simulink model "config5sim_KinematicController_PosCon_H1N4_H2N3"  (R2019b)
settings: Solver=ode4  StartTime=0.0  StopTime=60  FixedStep=0.01  RelTol=1e-3  EnableMultiTasking=on
InitFcn:
  | U_Path
  | roboparam
  | W_init = W_i;
  | 
  | xref_min = min(x_ref);
  | xref_max = max(x_ref);
  | yref_min = min(y_ref);
  | yref_max = max(y_ref);
  | 
  | xQ_min = min(xQ);
  | xQ_max = max(xQ);
  | yQ_min = min(yQ);
  | yQ_max = max(yQ);
  | 
  | xref_rng = xref_max - xref_min;
  | yref_rng = yref_max - yref_min;
  | xQ_rng = (xQ_max - yQ_min);
  | yQ_rng = (yQ_max - xQ_min);
  | 
  | xref_mean = mean(x_ref);
  | yref_mean = mean(y_ref);
  | xQ_mean = mean(xQ);
  | yQ_mean = mean(yQ);
  | 
  | xref_std = sqrt(var(x_ref));
  | yref_std = sqrt(var(y_ref));
  | xQ_std = sqrt(var(xQ));
  | yQ_std = sqrt(var(yQ));
StopFcn:
  | figure(1)
  | plot(xyref.DATA(:,1),xyref.DATA(:,2),'--black')
  | hold on
  | plot(xy_axon.DATA(:,1),xy_axon.DATA(:,2),'red')
  | hold on
  | plot(xy_trolley.DATA(:,1),xy_trolley.DATA(:,2),'green')
  | legend('Reference trajectory', 'Robot trajectory', 'Trailer trajectory')
  | 
  | figure(2)
  | plot(tq, errorX(:,1),'-red')
  | hold on
  | plot(tq, errorY(:,1),'-green')
  | hold on
  | legend('Error Linear', 'Error Angular')
values from neighbouring files (symbols this model uses):
  L = 0.387/2    (= 0.1935)    [roboparam.m]
  psicw10 = 0    [roboparam.m]
  psicw20 = 0    [roboparam.m]
  psicw30 = 0    [roboparam.m]
  psicw40 = 0    [roboparam.m]
  rho0 = 0.5    [roboparam.m]
  rho1 = 1    [roboparam.m]
  rhoH = 0.075    [roboparam.m]
  th0 = 0*pi/180    (= 0)    [roboparam.m]
  th1 = 0*pi/180    (= 0)    [roboparam.m]
  v0 = 0    [roboparam.m]
  w0 = 0    [roboparam.m]
  W_i = W_out(end,:)    [Looper4Neurons.m]    (also in Looper4NeuronsXY.m; LooperManualNet.m)
  xaxon0 = xtrolley0+rho1*cos(th1)+rho0*cos(th0)    [roboparam.m]
  xtrolley0 = -1.5    [roboparam.m]
  yaxon0 = ytrolley0+rho1*sin(th1)+rho0*sin(th0)    [roboparam.m]
  ytrolley0 = -0.75    [roboparam.m]
undefined symbols (not defined in the file or in its folder): sigbuilder_block
libraries: neural x76, simulink x2
(part 1 of 2)
settings Model: Creator=e0010448  LastModifiedBy=vladkhon
settings SolverCC: AlgebraicLoopSolver=LineSearch
settings DataIOCC: LimitDataPoints=on  SaveFormat=StructureWithTime  SignalLogging=off  DSMLogging=off  ReturnWorkspaceOutputs=off
settings OptimizationCC: BlockReduction=off  BufferReuse=off  LifeSpan=inf
settings DebuggingCC: AlgebraicLoopMsg=none  UnconnectedInputMsg=none  UnconnectedOutputMsg=none  UnconnectedLineMsg=none  AllowSymbolicDim=off  SFUnexpectedBacktrackingDiag=warning  SFNoUnconditionalDefaultTransitionDiag=warning  SFExecutionAtInitializationDiag=none  ArithmeticOperatorsInVariantConditions=warning
settings HardwareCC: ProdBitPerPointer=32  ProdBitPerSizeT=32  ProdBitPerPtrDiffT=32  ProdLargestAtomicFloat=None  ProdIntDivRoundTo=Undefined  ProdEndianess=Unspecified  ProdWordSize=32  ProdHWDeviceType=32-bit Generic
settings ModelReferenceCC: PropagateSignalLabelsOutOfModel=off
settings SFSimCC: SimUseLocalCustomCode=off  SimParseCustomCode=off  CustomCodeUndefinedFunction=UseInterfaceOnly
settings RTWCC: RTWUseLocalCustomCode=off
settings CodeAppCC: StateflowObjectComments=on
settings GRTTargetCC: TargetLangStandard=C89/C90 (ANSI)  GeneratePreprocessorConditionals=Disable all
settings ConfigComp: CovMetricSettings=dw  CovHtmlReporting=on  CovSaveCumulativeToWorkspaceVar=on  CovSaveSingleToWorkspaceVar=on  CovExternalEMLEnable=off

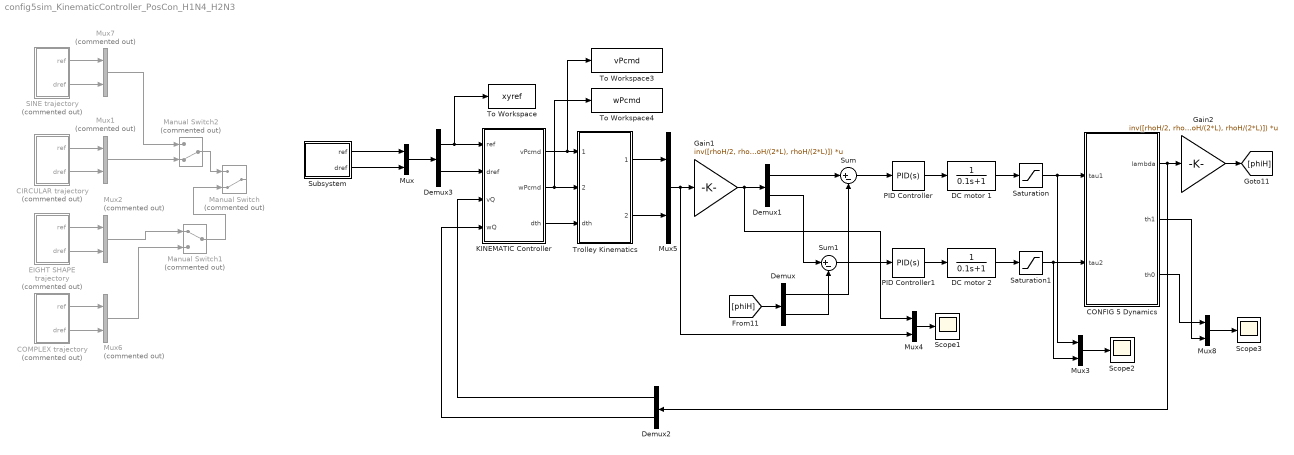
== system config5sim_KinematicController_PosCon_H1N4_H2N3 ==
  CIRCULAR trajectory : Subsystem  Commented=on
  COMPLEX trajectory : Subsystem  Commented=on
  CONFIG 5 Dynamics : Subsystem
  DC motor 1 : TransferFcn  Denominator=[0.1 1]
  DC motor 2 : TransferFcn  Denominator=[0.1 1]
  Demux{,1..3} (4 alike) : Demux  Outputs=2
  EIGHT SHAPE trajectory : Subsystem  Commented=on
  Gain1 : Gain  Gain=inv([rhoH/2, rhoH/2; -rhoH/(2*L), rhoH/(2*L)])  Multiplication=Matrix(K*u)
  Gain2 : Gain  Gain=inv([rhoH/2, rhoH/2; -rhoH/(2*L), rhoH/(2*L)])  Multiplication=Matrix(K*u)
  KINEMATIC Controller : Subsystem
  Manual Switch : ManualSwitch  Commented=on  CurrentSetting=0
  Manual Switch1 : ManualSwitch  Commented=on
  Manual Switch2 : ManualSwitch  Commented=on  CurrentSetting=0
  Mux{,3..5,8} (5 alike) : Mux  Inputs=2
  Mux{1..2,6..7} (4 alike) : Mux  Commented=on  Inputs=2
  PID Controller : simulink/Continuous/PID Controller  Controller=PID  Form=Parallel  TimeDomain=Continuous-time  SampleTime=-1  IntegratorMethod=Forward Euler  FilterMethod=Forward Euler  ControllerParametersSource=internal  P=3  I=5  D=1  UseFilter=on  N=100  TunerSelectOption=Transfer Function Based (PID Tuner App)  InitialConditionSource=internal  InitialConditionForIntegrator=0  InitialConditionForFilter=0  DifferentiatorICPrevScaledInput=0  ExternalReset=none  TrackingMode=off  Kt=1  LimitOutput=off  UpperSaturationLimit=inf  LowerSaturationLimit=-inf  LinearizeAsGain=on  AntiWindupMode=none  Kb=1  POutMin=[]  POutMax=[]  IOutMin=[]  IOutMax=[]  DOutMin=[]  DOutMax=[]  NOutMin=[]  NOutMax=[]  SumOutMin=[]  SumOutMax=[]  SaturationOutMin=[]  SaturationOutMax=[]  PParamMin=[]  PParamMax=[]  IParamMin=[]  IParamMax=[]  DParamMin=[]  DParamMax=[]  NParamMin=[]  NParamMax=[]  KbParamMin=[]  KbParamMax=[]  KtParamMin=[]  KtParamMax=[]  KbOutMin=[]  KbOutMax=[]  KtOutMin=[]  KtOutMax=[]  IntegratorOutMin=[]  IntegratorOutMax=[]  FilterOutMin=[]  FilterOutMax=[]  SumI1OutMin=[]  SumI1OutMax=[]  SumI2OutMin=[]  SumI2OutMax=[]  SumI3OutMin=[]  SumI3OutMax=[]  SumI4OutMin=[]  SumI4OutMax=[]  SumDOutMin=[]  SumDOutMax=[]  DifferentiatorOutMin=[]  DifferentiatorOutMax=[]  FilterDiffOutCoefMin=[]  FilterDiffOutCoefMax=[]  ReciprocalOutMin=[]  ReciprocalOutMax=[]  SumDenOutMin=[]  SumDenOutMax=[]  SumNumOutMin=[]  SumNumOutMax=[]  DivideOutMin=[]  DivideOutMax=[]  IntegratorContinuousStateAttributes=''  IntegratorStateMustResolveToSignalObject=off  IntegratorRTWStateStorageClass=Auto  FilterContinuousStateAttributes=''  FilterStateMustResolveToSignalObject=off  FilterRTWStateStorageClass=Auto  ParallelPVariant=InternalParameters  IdealPVariant=Disabled  IVariant=InternalParameters  DVariant=InternalParameters  IntegratorVariant=Continuous  SatVariant=Disabled  AWVariant=Passthrough  PCopyVariant=Disabled  TRVariant=Disabled  FdbkBlocksVariant=Forward  IdealPFdbkVariant=Disabled  SatFdbkVariant=Disabled  DerivativeFilterVariant=ContFilter  NVariant=InternalParameters  NCopyVariant=Disabled  FilterICVariant=InternalICsFilter  IntegratorICVariant=InternalICs  ExternalResetVariant=Disabled  TRSumVariant=Passthrough  SumFdbkVariant=Disabled  SumVariant=Sum_PID
  PID Controller1 : simulink/Continuous/PID Controller  Controller=PID  Form=Parallel  TimeDomain=Continuous-time  SampleTime=-1  IntegratorMethod=Forward Euler  FilterMethod=Forward Euler  ControllerParametersSource=internal  P=3  I=5  D=1  UseFilter=on  N=100  TunerSelectOption=Transfer Function Based (PID Tuner App)  InitialConditionSource=internal  InitialConditionForIntegrator=0  InitialConditionForFilter=0  DifferentiatorICPrevScaledInput=0  ExternalReset=none  TrackingMode=off  Kt=1  LimitOutput=off  UpperSaturationLimit=inf  LowerSaturationLimit=-inf  LinearizeAsGain=on  AntiWindupMode=none  Kb=1  POutMin=[]  POutMax=[]  IOutMin=[]  IOutMax=[]  DOutMin=[]  DOutMax=[]  NOutMin=[]  NOutMax=[]  SumOutMin=[]  SumOutMax=[]  SaturationOutMin=[]  SaturationOutMax=[]  PParamMin=[]  PParamMax=[]  IParamMin=[]  IParamMax=[]  DParamMin=[]  DParamMax=[]  NParamMin=[]  NParamMax=[]  KbParamMin=[]  KbParamMax=[]  KtParamMin=[]  KtParamMax=[]  KbOutMin=[]  KbOutMax=[]  KtOutMin=[]  KtOutMax=[]  IntegratorOutMin=[]  IntegratorOutMax=[]  FilterOutMin=[]  FilterOutMax=[]  SumI1OutMin=[]  SumI1OutMax=[]  SumI2OutMin=[]  SumI2OutMax=[]  SumI3OutMin=[]  SumI3OutMax=[]  SumI4OutMin=[]  SumI4OutMax=[]  SumDOutMin=[]  SumDOutMax=[]  DifferentiatorOutMin=[]  DifferentiatorOutMax=[]  FilterDiffOutCoefMin=[]  FilterDiffOutCoefMax=[]  ReciprocalOutMin=[]  ReciprocalOutMax=[]  SumDenOutMin=[]  SumDenOutMax=[]  SumNumOutMin=[]  SumNumOutMax=[]  DivideOutMin=[]  DivideOutMax=[]  IntegratorContinuousStateAttributes=''  IntegratorStateMustResolveToSignalObject=off  IntegratorRTWStateStorageClass=Auto  FilterContinuousStateAttributes=''  FilterStateMustResolveToSignalObject=off  FilterRTWStateStorageClass=Auto  ParallelPVariant=InternalParameters  IdealPVariant=Disabled  IVariant=InternalParameters  DVariant=InternalParameters  IntegratorVariant=Continuous  SatVariant=Disabled  AWVariant=Passthrough  PCopyVariant=Disabled  TRVariant=Disabled  FdbkBlocksVariant=Forward  IdealPFdbkVariant=Disabled  SatFdbkVariant=Disabled  DerivativeFilterVariant=ContFilter  NVariant=InternalParameters  NCopyVariant=Disabled  FilterICVariant=InternalICsFilter  IntegratorICVariant=InternalICs  ExternalResetVariant=Disabled  TRSumVariant=Passthrough  SumFdbkVariant=Disabled  SumVariant=Sum_PID
  SINE trajectory : Subsystem  Commented=on
  Saturation : Saturate  UpperLimit=40  LowerLimit=-40
  Saturation1 : Saturate  UpperLimit=40  LowerLimit=-40
  Scope1 : Scope
  Scope2 : Scope
  Scope3 : Scope
  Subsystem : Subsystem
  Sum : Sum  Inputs=|+-
  Sum1 : Sum  Inputs=|+-
  To Workspace : ToWorkspace  VariableName=xyref  SaveFormat=Timeseries  SampleTime=-1
  To Workspace3 : ToWorkspace  VariableName=vPcmd  SampleTime=-1
      settings: Save2DSignal=2-D array (concatenate along first dimension)
  To Workspace4 : ToWorkspace  VariableName=wPcmd  SampleTime=-1
      settings: Save2DSignal=2-D array (concatenate along first dimension)
  Trolley Kinematics : Subsystem
  wires:
  Sum/1 -> PID Controller/1
  CONFIG 5 Dynamics/1(lambda) -> Gain2/1, Demux2/1
  [phiH] -> Demux/1
  Demux/1 -> Sum/2
  Demux/2 -> Sum1/2
  Sum1/1 -> PID Controller1/1
  Mux4/1 -> Scope1/1
  Mux5/1 -> Mux4/2, Gain1/1
  Gain2/1 -> [phiH]
  Demux1/1 -> Sum/1
  Demux1/2 -> Sum1/1
  Mux3/1 -> Scope2/1
  Gain1/1 -> Mux4/1, Demux1/1
  PID Controller/1 -> DC motor 1/1
  PID Controller1/1 -> DC motor 2/1
  Demux2/1 -> KINEMATIC Controller/3(vQ)
  Demux2/2 -> KINEMATIC Controller/4(wQ)
  CIRCULAR trajectory/1(ref) -> Mux1/1
  CIRCULAR trajectory/2(dref) -> Mux1/2
  Demux3/1 -> To Workspace/1, KINEMATIC Controller/1(ref)
  Demux3/2 -> KINEMATIC Controller/2(dref)
  EIGHT SHAPE trajectory/1(ref) -> Mux2/1
  EIGHT SHAPE trajectory/2(dref) -> Mux2/2
  Mux2/1 -> Manual Switch1/1
  Manual Switch1/1 -> Manual Switch/2
  Mux6/1 -> Manual Switch1/2
  COMPLEX trajectory/1(ref) -> Mux6/1
  COMPLEX trajectory/2(dref) -> Mux6/2
  Manual Switch2/1 -> Manual Switch/1
  Mux1/1 -> Manual Switch2/2
  Mux7/1 -> Manual Switch2/1
  SINE trajectory/1(ref) -> Mux7/1
  SINE trajectory/2(dref) -> Mux7/2
  DC motor 1/1 -> Saturation/1
  Saturation/1 -> Mux3/1, CONFIG 5 Dynamics/1(tau1)
  DC motor 2/1 -> Saturation1/1
  Saturation1/1 -> Mux3/2, CONFIG 5 Dynamics/2(tau2)
  KINEMATIC Controller/1(vPcmd) -> To Workspace3/1, Trolley Kinematics/1(vPcmd)
  KINEMATIC Controller/2(wPcmd) -> Trolley Kinematics/2(wPcmd), To Workspace4/1
  Trolley Kinematics/1(vQcmd) -> Mux5/1
  Trolley Kinematics/2(wQcmd) -> Mux5/2
  KINEMATIC Controller/3(dth) -> Trolley Kinematics/3(dth)
  Mux8/1 -> Scope3/1
  CONFIG 5 Dynamics/2(th1) -> Mux8/2
  CONFIG 5 Dynamics/3(th0) -> Mux8/1
  Subsystem/2("dref ") -> Mux/2
  Subsystem/1(ref) -> Mux/1
  Mux/1 -> Demux3/1

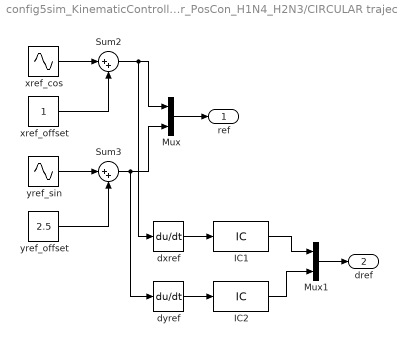
== system config5sim_KinematicController_PosCon_H1N4_H2N3/CIRCULAR trajectory ==
  IC1 : InitialCondition  Value=0
  IC2 : InitialCondition  Value=7.5*0.05
  Mux : Mux  Inputs=2
  Mux1 : Mux  Inputs=2
  Sum2 : Sum  Inputs=|++
  Sum3 : Sum  Inputs=|++
  dxref : Derivative  CoefficientInTFapproximation=100
  dyref : Derivative  CoefficientInTFapproximation=100
  xref_cos : Sin  Amplitude=25  Frequency=0.05  Phase=pi/2  Samples=100  SampleTime=0  Offset=10
  xref_offset : Constant
  yref_offset : Constant  Value=2.5
  yref_sin : Sin  Amplitude=25  Frequency=0.05  Samples=100  SampleTime=0  Offset=10
  ref : Outport  VectorParamsAs1DForOutWhenUnconnected=off
  dref : Outport  Port=2  VectorParamsAs1DForOutWhenUnconnected=off
  wires:
  xref_cos/1 -> Sum2/1
  yref_sin/1 -> Sum3/1
  xref_offset/1 -> Sum2/2
  Sum2/1 -> dxref/1, Mux/1
  yref_offset/1 -> Sum3/2
  Sum3/1 -> dyref/1, Mux/2
  Mux/1 -> ref/1
  dxref/1 -> IC1/1
  dyref/1 -> IC2/1
  IC2/1 -> Mux1/2
  IC1/1 -> Mux1/1
  Mux1/1 -> dref/1

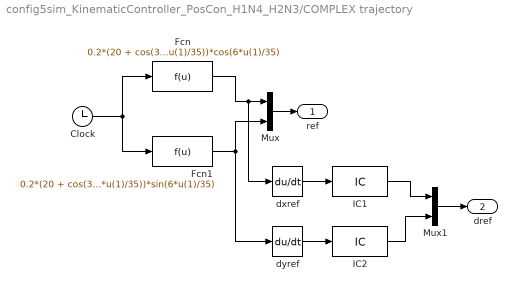
== system config5sim_KinematicController_PosCon_H1N4_H2N3/COMPLEX trajectory ==
  Clock : Clock
  Fcn : Fcn  Expr=0.2*(20 + cos(36*u(1)/35))*cos(6*u(1)/35)
  Fcn1 : Fcn  Expr=0.2*(20 + cos(36*u(1)/35))*sin(6*u(1)/35)
  IC1 : InitialCondition  Value=0
  IC2 : InitialCondition  Value=18*0.2/5
  Mux : Mux  Inputs=2
  Mux1 : Mux  Inputs=2
  dxref : Derivative  CoefficientInTFapproximation=100
  dyref : Derivative  CoefficientInTFapproximation=100
  ref : Outport  VectorParamsAs1DForOutWhenUnconnected=off
  dref : Outport  Port=2  VectorParamsAs1DForOutWhenUnconnected=off
  wires:
  Clock/1 -> Fcn1/1, Fcn/1
  Mux/1 -> ref/1
  dxref/1 -> IC1/1
  dyref/1 -> IC2/1
  IC2/1 -> Mux1/2
  IC1/1 -> Mux1/1
  Mux1/1 -> dref/1
  Fcn/1 -> dxref/1, Mux/1
  Fcn1/1 -> dyref/1, Mux/2

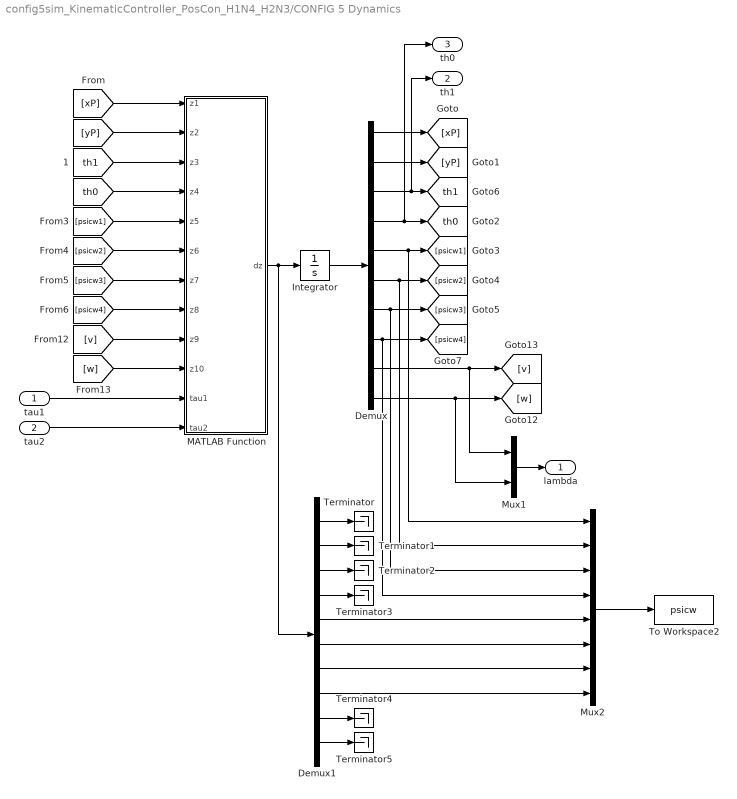
== system config5sim_KinematicController_PosCon_H1N4_H2N3/CONFIG 5 Dynamics ==
  tau1 : Inport
  tau2 : Inport  Port=2
  Demux : Demux  Outputs=10
  Demux1 : Demux  Outputs=10
  Integrator : Integrator  InitialCondition=[xtrolley0 ytrolley0 th1 th0 psicw10 psicw20 psicw30 psicw40 v0 w0]
  MATLAB Function : MATLAB Function  TreatAsAtomicUnit=on
  Mux1 : Mux  Inputs=2
  Mux2 : Mux  Inputs=8
  Terminator{,1..5} (6 alike) : Terminator
  To Workspace2 : ToWorkspace  VariableName=psicw  SaveFormat=Timeseries  SampleTime=-1
  lambda : Outport  VectorParamsAs1DForOutWhenUnconnected=off
  th1 : Outport  Port=2  VectorParamsAs1DForOutWhenUnconnected=off
  th0 : Outport  Port=3  VectorParamsAs1DForOutWhenUnconnected=off
  tag scope: th0=global, th1=global
  wires:
  Mux1/1 -> lambda/1
  Integrator/1 -> Demux/1
  Demux/10 -> Mux1/2, [w]
  Demux/9 -> Mux1/1, [v]
  Demux/8 -> [psicw4], Mux2/4
  Demux/7 -> [psicw3], Mux2/3
  Demux/6 -> [psicw2], Mux2/2
  Demux/5 -> [psicw1], Mux2/1
  Demux/2 -> [yP]
  Demux/1 -> [xP]
  MATLAB Function/1(dz) -> Demux1/1, Integrator/1
  [xP] -> MATLAB Function/1(z1)
  [yP] -> MATLAB Function/2(z2)
  [psicw1] -> MATLAB Function/5(z5)
  [psicw2] -> MATLAB Function/6(z6)
  [psicw3] -> MATLAB Function/7(z7)
  [psicw4] -> MATLAB Function/8(z8)
  [v] -> MATLAB Function/9(z9)
  [w] -> MATLAB Function/10(z10)
  [th1] -> MATLAB Function/3(z3)
  [th0] -> MATLAB Function/4(z4)
  Demux/3 -> th1/1, [th1]
  Demux/4 -> th0/1, [th0]
  tau1/1 -> MATLAB Function/11(tau1)
  tau2/1 -> MATLAB Function/12(tau2)
  Demux1/8 -> Mux2/8
  Demux1/7 -> Mux2/7
  Demux1/6 -> Mux2/6
  Demux1/5 -> Mux2/5
  Mux2/1 -> To Workspace2/1
  Demux1/1 -> Terminator/1
  Demux1/2 -> Terminator1/1
  Demux1/4 -> Terminator3/1
  Demux1/3 -> Terminator2/1
  Demux1/10 -> Terminator5/1
  Demux1/9 -> Terminator4/1

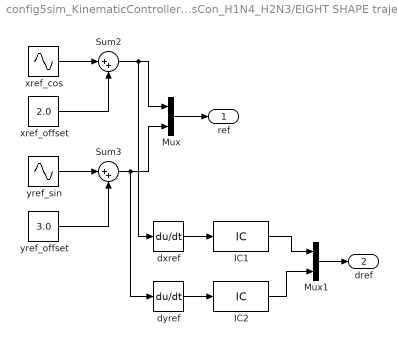
== system config5sim_KinematicController_PosCon_H1N4_H2N3/EIGHT SHAPE trajectory ==
  IC1 : InitialCondition  Value=2*0.1
  IC2 : InitialCondition  Value=2*0.05
  Mux : Mux  Inputs=2
  Mux1 : Mux  Inputs=2
  Sum2 : Sum  Inputs=|++
  Sum3 : Sum  Inputs=|++
  dxref : Derivative  CoefficientInTFapproximation=100
  dyref : Derivative  CoefficientInTFapproximation=100
  xref_cos : Sin  Amplitude=2  Frequency=0.1  Samples=100  SampleTime=0  Offset=10
  xref_offset : Constant  Value=2.0
  yref_offset : Constant  Value=3.0
  yref_sin : Sin  Amplitude=2  Frequency=0.05  Samples=100  SampleTime=0  Offset=10
  ref : Outport  VectorParamsAs1DForOutWhenUnconnected=off
  dref : Outport  Port=2  VectorParamsAs1DForOutWhenUnconnected=off
  wires:
  xref_cos/1 -> Sum2/1
  yref_sin/1 -> Sum3/1
  xref_offset/1 -> Sum2/2
  yref_offset/1 -> Sum3/2
  Sum2/1 -> dxref/1, Mux/1
  Sum3/1 -> dyref/1, Mux/2
  Mux/1 -> ref/1
  dxref/1 -> IC1/1
  dyref/1 -> IC2/1
  IC2/1 -> Mux1/2
  IC1/1 -> Mux1/1
  Mux1/1 -> dref/1

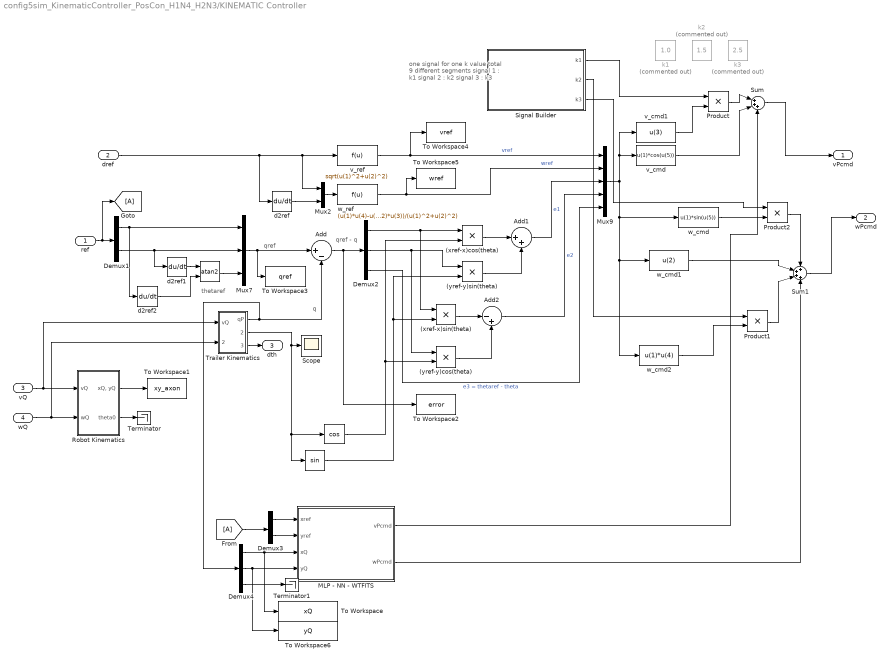
== system config5sim_KinematicController_PosCon_H1N4_H2N3/KINEMATIC Controller ==
  note: one signal for one k value
      | total 9 different segments
      |
      | signal 1 : k1
      | signal 2 : k2
      | signal 3 : k3
  note: qref - q
  note: q
  note: qref
  note: thetaref
  ref : Inport
  dref : Inport  Port=2
  vQ : Inport  Port=3
  wQ : Inport  Port=4
  "     " : Trigonometry  Operator=atan2
  "         " : Trigonometry  Operator=cos
  "          " : Trigonometry
  (xref-x)cos(theta) : Product
  (xref-x)sin(theta) : Product
  (yref-y)cos(theta) : Product
  (yref-y)sin(theta) : Product
  Add : Sum  Inputs=|+-
  Add1 : Sum  Inputs=|++
  Add2 : Sum  Inputs=|-+
  Demux1 : Demux  Outputs=2
  Demux2 : Demux  Outputs=3
  Demux3 : Demux  Outputs=2
  Demux4 : Demux  Outputs=3
  MLP - NN - WTFITS : Subsystem
  Mux2 : Mux  Inputs=2
  Mux7 : Mux  Inputs=3
  Mux9 : Mux  Inputs=5
  Product : Product
  Product1 : Product
  Product2 : Product
  Robot Kinematics : Subsystem
  Scope : Scope
  Signal Builder : Subsystem  Tag=STV Subsys  LoadFcn=sigbuilder_block('load');  StartFcn=sigbuilder_block('start');  StopFcn=sigbuilder_block('stop');  ClipboardFcn=sigbuilder_block('clipboard');  mask(Sigbuilder block){tuvar=[0:10]}
      mask help: Simulink:masks:SigbuilderBlock_MD
      mask init:
      | if ~strcmp(get_param(bdroot(gcbh),'SimulationStatus'),'stopped') tuvar = sigbuilder_block('maskInit'); end
      settings: CopyFcn=sigbuilder_block('copy');  DeleteFcn=sigbuilder_block('delete');  ModelCloseFcn=sigbuilder_block('modelClose');  PreSaveFcn=sigbuilder_block('preSave');  PauseFcn=sigbuilder_block('pause');  ContinueFcn=sigbuilder_block('continue');  NameChangeFcn=sigbuilder_block('namechange');  OpenFcn=sigbuilder_block('open',[5.5 55 949 418 ]);  CloseFcn=sigbuilder_block('close');
      mask Display: plot(0, 0, 100, 100,[2, 2, 32, 32, 2], [68, 8, 8, 68, 68],[32, 2], [38, 38], [32, 19, 2],[53, 60, 44], [32, 17, 17, 2],[16, 16, 31, 31]);txt = getActiveGroup(gcbh);text(2, 100, txt,'verticalAlignment', 'top');
  Sum : Sum  Inputs=|+++
  Sum1 : Sum  Inputs=++++
  Terminator : Terminator
  Terminator1 : Terminator
  To Workspace : ToWorkspace  VariableName=xQ  SaveFormat=Timeseries  SampleTime=-1
  To Workspace1 : ToWorkspace  VariableName=xy_axon  SaveFormat=Timeseries  SampleTime=-1
  To Workspace2 : ToWorkspace  VariableName=error  SampleTime=-1
  To Workspace3 : ToWorkspace  VariableName=qref  SampleTime=-1
  To Workspace4 : ToWorkspace  VariableName=vref  SampleTime=-1
  To Workspace5 : ToWorkspace  VariableName=wref  SampleTime=-1
  To Workspace6 : ToWorkspace  VariableName=yQ  SaveFormat=Timeseries  SampleTime=-1
  Trailer Kinematics : Subsystem
  d2ref : Derivative  CoefficientInTFapproximation=100
  d2ref1 : Derivative  CoefficientInTFapproximation=100
  d2ref2 : Derivative  CoefficientInTFapproximation=100
  "k1 " : Constant  Commented=on  Value=1.0
  "k2 " : Constant  Commented=on  Value=1.5
  "k3 " : Constant  Commented=on  Value=2.5
  v_cmd : Fcn  Expr=u(1)*cos(u(5))
  v_cmd1 : Fcn  Expr=u(3)
  v_ref : Fcn  Expr=sqrt(u(1)^2+u(2)^2)
  w_cmd : Fcn  Expr=u(1)*sin(u(5))
  w_cmd1 : Fcn  Expr=u(2)
  w_cmd2 : Fcn  Expr=u(1)*u(4)
  w_ref : Fcn  Expr=(u(1)*u(4)-u(2)*u(3))/(u(1)^2+u(2)^2)
  vPcmd : Outport  VectorParamsAs1DForOutWhenUnconnected=off
  wPcmd : Outport  Port=2  VectorParamsAs1DForOutWhenUnconnected=off
  dth : Outport  Port=3  VectorParamsAs1DForOutWhenUnconnected=off
  wires:
  (xref-x)sin(theta)/1 -> Add2/1
  (yref-y)cos(theta)/1 -> Add2/2
  v_ref/1 -> To Workspace4/1, Mux9/1  "vref"
  w_ref/1 -> To Workspace5/1, Mux9/2  "wref"
  Add/1 -> To Workspace2/1, Demux2/1
  Mux2/1 -> w_ref/1
  dref/1 -> d2ref/1, Mux2/1, v_ref/1
  d2ref/1 -> Mux2/2
  Mux7/1 -> To Workspace3/1, Add/1
  Demux2/1 -> (xref-x)sin(theta)/1, (xref-x)cos(theta)/1
  (xref-x)cos(theta)/1 -> Add1/1
  (yref-y)sin(theta)/1 -> Add1/2
  Add1/1 -> Mux9/3  "e1"
  Add2/1 -> Mux9/4  "e2"
  Demux2/3 -> Mux9/5  "e3 = thetaref - theta"
  Demux2/2 -> (yref-y)cos(theta)/1, (yref-y)sin(theta)/1
  "         "/1 -> (yref-y)cos(theta)/2, (xref-x)cos(theta)/2
  "          "/1 -> (xref-x)sin(theta)/2, (yref-y)sin(theta)/2
  Mux9/1 -> w_cmd/1, w_cmd2/1, w_cmd1/1, v_cmd1/1, v_cmd/1
  ref/1 -> [A], Demux1/1
  Demux1/1 -> Mux7/1, d2ref2/1
  Demux1/2 -> d2ref1/1, Mux7/2
  "     "/1 -> Mux7/3
  vQ/1 -> Trailer Kinematics/1(vQ), Robot Kinematics/1(vQ)
  wQ/1 -> Trailer Kinematics/2(wQ), Robot Kinematics/2(wQ)
  Robot Kinematics/1("xQ, yQ") -> To Workspace1/1
  Trailer Kinematics/1(qP) -> Demux4/1, Add/2
  Trailer Kinematics/3(dth) -> dth/1
  Trailer Kinematics/2(theta1) -> "         "/1, "          "/1, Scope/1
  d2ref1/1 -> "     "/1
  d2ref2/1 -> "     "/2
  Robot Kinematics/2(theta0) -> Terminator/1
  v_cmd1/1 -> Product/2
  Sum/1 -> vPcmd/1
  w_cmd2/1 -> Product1/2
  Sum1/1 -> wPcmd/1
  w_cmd/1 -> Product2/2
  Signal Builder/1(k1) -> Product/1
  Signal Builder/2(k2) -> Product1/1
  Signal Builder/3(k3) -> Product2/1
  MLP - NN - WTFITS/1(vPcmd) -> Sum/3
  MLP - NN - WTFITS/2(wPcmd) -> Sum1/4
  Demux3/1 -> MLP - NN - WTFITS/1("xref ")
  Demux3/2 -> MLP - NN - WTFITS/2(yref)
  Demux4/1 -> To Workspace/1, MLP - NN - WTFITS/3(xQ)
  Demux4/2 -> To Workspace6/1, MLP - NN - WTFITS/4(yQ)
  Product2/1 -> Sum1/1
  w_cmd1/1 -> Sum1/2
  Product1/1 -> Sum1/3
  Product/1 -> Sum/1
  v_cmd/1 -> Sum/2
  [A] -> Demux3/1
  Demux4/3 -> Terminator1/1

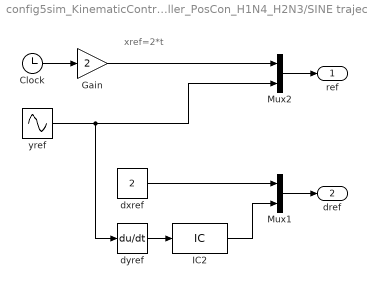
== system config5sim_KinematicController_PosCon_H1N4_H2N3/SINE trajectory ==
  note: xref=2*t
  Clock : Clock
  Gain : Gain  Gain=2
  IC2 : InitialCondition  Value=2*0.25
  Mux1 : Mux  Inputs=2
  Mux2 : Mux  Inputs=2
  dxref : Constant  Value=2
  dyref : Derivative  CoefficientInTFapproximation=100
  yref : Sin  Amplitude=2  Frequency=0.25  Samples=100  SampleTime=0  Offset=10
  ref : Outport  VectorParamsAs1DForOutWhenUnconnected=off
  dref : Outport  Port=2  VectorParamsAs1DForOutWhenUnconnected=off
  wires:
  yref/1 -> Mux2/2, dyref/1
  dyref/1 -> IC2/1
  IC2/1 -> Mux1/2
  dxref/1 -> Mux1/1
  Mux1/1 -> dref/1
  Mux2/1 -> ref/1
  Gain/1 -> Mux2/1
  Clock/1 -> Gain/1

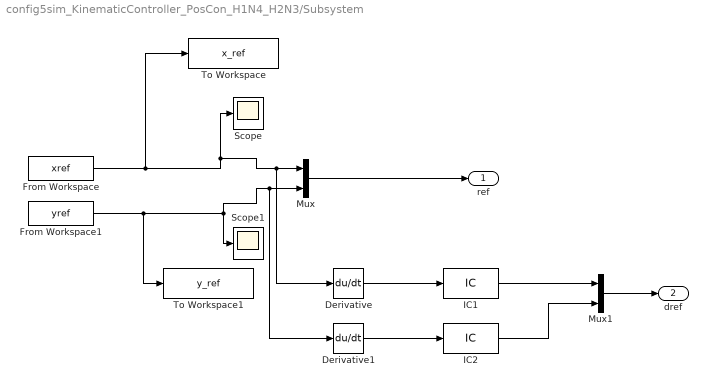
== system config5sim_KinematicController_PosCon_H1N4_H2N3/Subsystem ==
  Derivative : Derivative
  Derivative1 : Derivative
  From Workspace : FromWorkspace  VariableName=xref  SampleTime=0
  From Workspace1 : FromWorkspace  VariableName=yref  SampleTime=0
  IC1 : InitialCondition  Value=0
  IC2 : InitialCondition  Value=0.0001
  Mux : Mux  Inputs=2
  Mux1 : Mux  Inputs=2
  Scope : Scope
  Scope1 : Scope
  To Workspace : ToWorkspace  VariableName=x_ref  SampleTime=-1
  To Workspace1 : ToWorkspace  VariableName=y_ref  SampleTime=-1
  ref : Outport  VectorParamsAs1DForOutWhenUnconnected=off
  "dref " : Outport  Port=2  VectorParamsAs1DForOutWhenUnconnected=off
  wires:
  Mux/1 -> ref/1
  From Workspace/1 -> To Workspace/1, Scope/1, Derivative/1, Mux/1
  From Workspace1/1 -> Derivative1/1, Mux/2, Scope1/1, To Workspace1/1
  Mux1/1 -> "dref "/1
  Derivative/1 -> IC1/1
  Derivative1/1 -> IC2/1
  IC1/1 -> Mux1/1
  IC2/1 -> Mux1/2

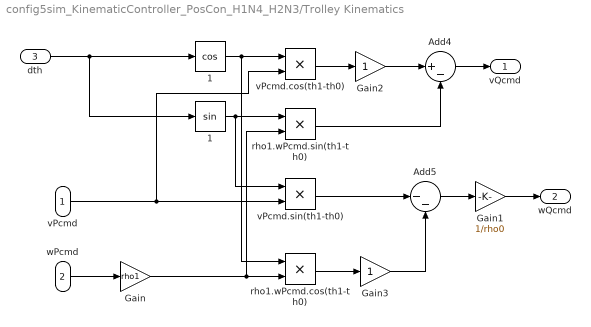
== system config5sim_KinematicController_PosCon_H1N4_H2N3/Trolley Kinematics ==
  vPcmd : Inport
  wPcmd : Inport  Port=2
  dth : Inport  Port=3
  "          1" : Trigonometry
  "         1" : Trigonometry  Operator=cos
  Add4 : Sum  Inputs=|+-
  Add5 : Sum  Inputs=|--
  Gain : Gain  Gain=rho1
  Gain1 : Gain  Gain=1/rho0
  Gain2 : Gain
  Gain3 : Gain
  rho1.wPcmd.cos(th1-th0) : Product
  rho1.wPcmd.sin(th1-th0) : Product
  vPcmd.cos(th1-th0) : Product
  vPcmd.sin(th1-th0) : Product
  vQcmd : Outport  VectorParamsAs1DForOutWhenUnconnected=off
  wQcmd : Outport  Port=2  VectorParamsAs1DForOutWhenUnconnected=off
  wires:
  "         1"/1 -> rho1.wPcmd.cos(th1-th0)/1, vPcmd.cos(th1-th0)/1
  dth/1 -> "         1"/1, "          1"/1
  "          1"/1 -> vPcmd.sin(th1-th0)/1, rho1.wPcmd.sin(th1-th0)/1
  Gain/1 -> rho1.wPcmd.sin(th1-th0)/2, rho1.wPcmd.cos(th1-th0)/2
  rho1.wPcmd.sin(th1-th0)/1 -> Add4/2
  vPcmd/1 -> vPcmd.cos(th1-th0)/2, vPcmd.sin(th1-th0)/2
  wPcmd/1 -> Gain/1
  Add5/1 -> Gain1/1
  Gain1/1 -> wQcmd/1
  vPcmd.sin(th1-th0)/1 -> Add5/1
  Add4/1 -> vQcmd/1
  vPcmd.cos(th1-th0)/1 -> Gain2/1
  Gain2/1 -> Add4/1
  rho1.wPcmd.cos(th1-th0)/1 -> Gain3/1
  Gain3/1 -> Add5/2

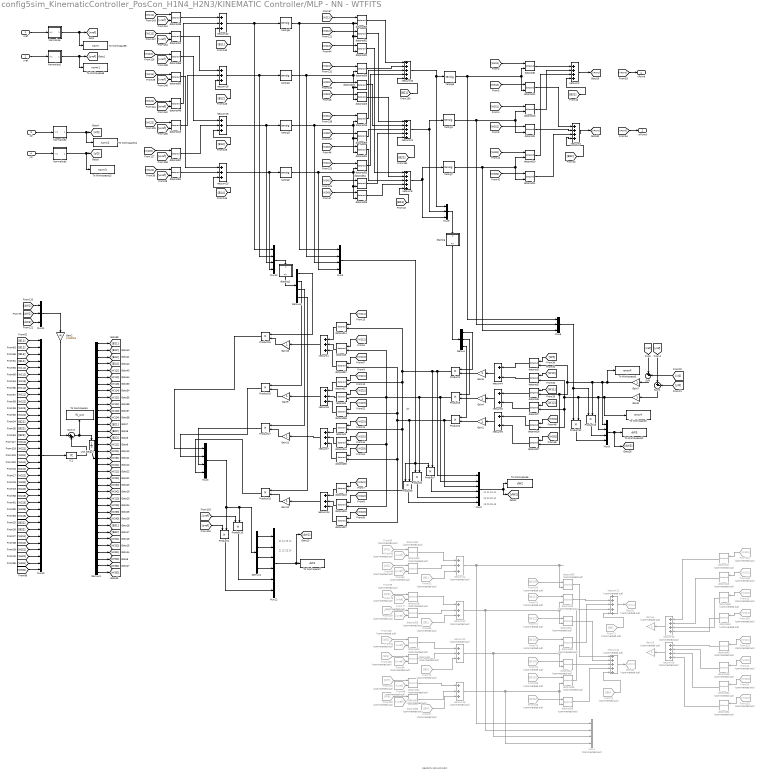
== system config5sim_KinematicController_PosCon_H1N4_H2N3/KINEMATIC Controller/MLP - NN - WTFITS ==
  note: NEURON GRAVEYARD
  note: 11 21 31 41
  note: 11 12 13 14
  note: del
  note: 21 22 23 24
  note: 12 22 32 42
  note: 13 23 33 43
  "xref " : Inport
  yref : Inport  Port=2
  xQ : Inport  Port=3
  yQ : Inport  Port=4
  Demux : Demux  Outputs=3
  Demux1 : Demux
  Demux3 : Demux  Outputs=35
  Demux4 : Demux
  From{77,80,94,100} (4 alike) : From  Commented=on  GotoTag=wref
  From101 : From  Commented=on  GotoTag=W7
  From102 : From  Commented=on  GotoTag=W8
  From104 : From  Commented=on  GotoTag=W10
  From105 : From  Commented=on  GotoTag=W15
  From106 : From  Commented=on  GotoTag=W16
  From107 : From  Commented=on  GotoTag=W4
  From108 : From  Commented=on  GotoTag=W5
  From109 : From  Commented=on  GotoTag=W6
  From112 : From  Commented=on  GotoTag=W111
  From113 : From  Commented=on  GotoTag=W121
  From148 : From  Commented=on  GotoTag=W112
  From150 : From  Commented=on  GotoTag=W114
  From151 : From  Commented=on  GotoTag=W124
  From22 : From  Commented=on  GotoTag=W122
  From23 : From  Commented=on  GotoTag=W113
  From24 : From  Commented=on  GotoTag=W123
  From69 : From  Commented=on  GotoTag=B1
  From70 : From  Commented=on  GotoTag=B3
  From71 : From  Commented=on  GotoTag=B5
  From72 : From  Commented=on  GotoTag=B6
  From73 : From  Commented=on  GotoTag=W11
  From74 : From  Commented=on  GotoTag=W12
  From{76,91,93,98} (4 alike) : From  Commented=on  GotoTag=vref
  From78 : From  Commented=on  GotoTag=W13
  From79 : From  Commented=on  GotoTag=W14
  From92 : From  Commented=on  GotoTag=B1
  From95 : From  Commented=on  GotoTag=W1
  From96 : From  Commented=on  GotoTag=W2
  From97 : From  Commented=on  GotoTag=B4
  From99 : From  Commented=on  GotoTag=W3
  Gain{1,4..5,7..12} (9 alike) : Gain
  Gain13 : Gain  Commented=on
  Gain14 : Gain  Commented=on
  Gain2 : Gain  Gain=0.000001
  Goto31 : Goto  Commented=on  GotoTag=vPcmd
  Goto32 : Goto  Commented=on  GotoTag=wPcmd
  IC1 : InitialCondition  Value=W_init
  Mux10 : Mux  Inputs=35
  Mux11 : Mux  Inputs=3
  Mux12 : Mux  Inputs=6
  Mux{3,5,8,13} (4 alike) : Mux
  Mux2 : Mux  Inputs=6
  Mux4 : Mux  Commented=on
  Mux6 : Mux  Inputs=3
  Mux9 : Mux  Inputs=3
  Normalise : Subsystem
  Normalise1 : Subsystem
  Normalise2 : Subsystem
  Normalise3 : Subsystem
  Product{1..7,10,12..13,15..18} (14 alike) : Product
  Sum : Sum  Inputs=|+-
  Sum1 : Sum  Inputs=|+-
  Sum17 : Sum  Inputs=|++
  To Workspace1 : ToWorkspace  VariableName=W_out  SampleTime=-1
  To Workspace11 : ToWorkspace  VariableName=norm2  SampleTime=-1
  To Workspace12 : ToWorkspace  VariableName=dW3  SampleTime=-1
  To Workspace13 : ToWorkspace  VariableName=norm3  SampleTime=-1
  To Workspace2 : ToWorkspace  VariableName=errorY  SampleTime=-1
  To Workspace3 : ToWorkspace  VariableName=errorX  SampleTime=-1
  To Workspace5 : ToWorkspace  VariableName=dW2  SampleTime=-1
  To Workspace6 : ToWorkspace  VariableName=norm1  SampleTime=-1
  To Workspace7 : ToWorkspace  VariableName=dW1  SampleTime=-1
  To Workspace8 : ToWorkspace  VariableName=norm  SampleTime=-1
  Unit Delay1 : UnitDelay  SampleTime=-1  HasFrameUpgradeWarning=on
  dotprod{1..27,37,44,48..59,65..67} (44 alike) : neural/Weight Functions/dotprod
      settings: SourceProductName=Deep Learning Toolbox
  dotprod{28..36,38..43,45..47,60..64} (23 alike) : neural/Weight Functions/dotprod  Commented=on
      settings: SourceProductName=Deep Learning Toolbox
  dtansig : Subsystem
  dtansig1 : Subsystem
  netsum{1,6..7,18..19,22..24} (8 alike) : Sum  Inputs=3  SaturateOnIntegerOverflow=on  InputSameDT=on  OutDataTypeStr=Inherit: Same as first input
  netsum{10..11,14..15} (4 alike) : Sum  Commented=on  Inputs=3  SaturateOnIntegerOverflow=on  InputSameDT=on  OutDataTypeStr=Inherit: Same as first input
  netsum12 : Sum  Commented=on  Inputs=5  SaturateOnIntegerOverflow=on  InputSameDT=on  OutDataTypeStr=Inherit: Same as first input
  netsum13 : Sum  Commented=on  Inputs=5  SaturateOnIntegerOverflow=on  InputSameDT=on  OutDataTypeStr=Inherit: Same as first input
  netsum2 : Sum  Inputs=4  SaturateOnIntegerOverflow=on  InputSameDT=on  OutDataTypeStr=Inherit: Same as first input
  netsum20 : Sum  Inputs=5  SaturateOnIntegerOverflow=on  InputSameDT=on  OutDataTypeStr=Inherit: Same as first input
  netsum21 : Sum  Inputs=5  SaturateOnIntegerOverflow=on  InputSameDT=on  OutDataTypeStr=Inherit: Same as first input
  netsum25 : Sum  Commented=on  Inputs=4  SaturateOnIntegerOverflow=on  InputSameDT=on  OutDataTypeStr=Inherit: Same as first input
  netsum26 : Sum  Commented=on  Inputs=4  SaturateOnIntegerOverflow=on  InputSameDT=on  OutDataTypeStr=Inherit: Same as first input
  netsum3 : Sum  Inputs=4  SaturateOnIntegerOverflow=on  InputSameDT=on  OutDataTypeStr=Inherit: Same as first input
  netsum4 : Sum  Inputs=2  SaturateOnIntegerOverflow=on  InputSameDT=on  OutDataTypeStr=Inherit: Same as first input
  netsum5 : Sum  Inputs=2  SaturateOnIntegerOverflow=on  InputSameDT=on  OutDataTypeStr=Inherit: Same as first input
  netsum8 : Sum  Inputs=5  SaturateOnIntegerOverflow=on  InputSameDT=on  OutDataTypeStr=Inherit: Same as first input
  netsum9 : Sum  Inputs=2  SaturateOnIntegerOverflow=on  InputSameDT=on  OutDataTypeStr=Inherit: Same as first input
  tansig{1..7} (7 alike) : neural/Transfer Functions/tansig
      settings: SourceProductName=Deep Learning Toolbox
  vPcmd : Outport
  wPcmd : Outport  Port=2
  wires:
  [yQ] -> Sum1/2
  [xref] -> Sum/1
  [yref] -> Sum1/1
  [W12] -> dotprod7/1
  [W9] -> dotprod3/1
  [W10] -> dotprod2/1
  [W11] -> dotprod6/1
  [xQ] -> Sum/2
  [W312] -> dotprod11/1
  [W311] -> dotprod8/1
  [W321] -> dotprod10/1
  [W322] -> dotprod9/1
  Mux6/1 -> Product12/1, Product13/1
  Sum/1 -> Gain7/1
  Sum1/1 -> Gain8/1
  dotprod11/1 -> netsum3/1
  From93/1 -> dotprod32/2
  From108/1 -> dotprod40/1
  netsum10/1 -> Mux4/2, dotprod42/2, dotprod31/2
  From72/1 -> netsum13/5
  dotprod36/1 -> netsum13/1
  From77/1 -> dotprod29/2
  From80/1 -> dotprod41/2
  From73/1 -> dotprod42/1
  From74/1 -> dotprod31/1
  dotprod28/1 -> netsum10/1
  dotprod35/1 -> netsum15/2
  dotprod39/1 -> netsum12/4
  dotprod30/1 -> netsum12/3
  From96/1 -> dotprod33/1
  From78/1 -> dotprod30/1
  dotprod40/1 -> netsum11/1
  From109/1 -> dotprod41/1
  dotprod41/1 -> netsum11/2
  dotprod32/1 -> netsum14/1
  From99/1 -> dotprod28/1
  From107/1 -> dotprod29/1
  From79/1 -> dotprod43/1
  dotprod29/1 -> netsum10/2
  From92/1 -> netsum14/3
  From100/1 -> dotprod35/2
  netsum14/1 -> dotprod36/2, Mux4/1
  dotprod33/1 -> netsum14/2
  From69/1 -> netsum10/3
  From98/1 -> dotprod34/2
  From97/1 -> netsum15/3
  From102/1 -> dotprod35/1
  From95/1 -> dotprod32/1
  From91/1 -> dotprod40/2
  From101/1 -> dotprod34/1
  netsum11/1 -> Mux4/3, dotprod30/2, dotprod43/2
  dotprod34/1 -> netsum15/1
  From94/1 -> dotprod33/2
  dotprod43/1 -> netsum13/3
  From70/1 -> netsum11/3
  dotprod31/1 -> netsum13/2
  netsum15/1 -> Mux4/4, dotprod38/2, dotprod39/2
  From71/1 -> netsum12/5
  From105/1 -> dotprod39/1
  dotprod42/1 -> netsum12/2
  dotprod38/1 -> netsum13/4
  From104/1 -> dotprod36/1
  From76/1 -> dotprod28/2
  From106/1 -> dotprod38/1
  dotprod9/1 -> netsum3/2
  dotprod8/1 -> netsum2/1
  dotprod10/1 -> netsum2/2
  [vPcmd] -> vPcmd/1
  [wPcmd] -> wPcmd/1
  netsum13/1 -> Goto32/1
  netsum12/1 -> Goto31/1
  tansig1/1 -> dotprod9/2, dotprod10/2, Mux6/2
  tansig5/1 -> dotprod8/2, dotprod11/2, Mux6/1
  Mux9/1 -> dtansig/1(Z)
  dtansig/1(Phi) -> Demux/1
  Demux3/3 -> [B13]
  [W112] -> Mux10/6
  Mux11/1 -> Gain2/1
  Demux3/6 -> [W112]
  Demux3/2 -> [B12]
  Demux3/8 -> [W114]
  [dW2] -> Mux11/2
  Demux3/10 -> [W122]
  Demux3/11 -> [W123]
  Demux3/4 -> [B14]
  Demux3/9 -> [W121]
  Demux3/7 -> [W113]
  [W121] -> Mux10/9
  [W111] -> Mux10/5
  [W123] -> Mux10/11
  Demux3/5 -> [W111]
  [B13] -> Mux10/3
  Demux3/12 -> [W124]
  [W122] -> Mux10/10
  Demux3/1 -> [B11]
  [B12] -> Mux10/2
  [B11] -> Mux10/1
  [W114] -> Mux10/8
  [B14] -> Mux10/4
  [W113] -> Mux10/7
  [W124] -> Mux10/12
  IC1/1 -> Sum17/2
  netsum4/1 -> Gain5/1
  netsum5/1 -> Gain4/1
  Gain4/1 -> Product5/2
  Gain5/1 -> Product4/2
  dotprod6/1 -> netsum5/1
  dotprod7/1 -> netsum5/2
  Product4/1 -> Product7/2, dotprod17/2, dotprod16/2, dotprod1/2, dotprod14/2, Mux2/1
  Product5/1 -> Mux2/2, Product6/2, dotprod15/2, dotprod44/2, dotprod4/2, dotprod5/2
  [B21] -> Mux10/13
  [B22] -> Mux10/14
  [B23] -> Mux10/15
  [W211] -> Mux10/16
  [W221] -> Mux10/17
  [W231] -> Mux10/18
  Demux3/13 -> [B21]
  Demux3/14 -> [B22]
  Demux3/15 -> [B23]
  Demux3/16 -> [W211]
  Demux3/17 -> [W221]
  Demux3/18 -> [W231]
  [dW3] -> Mux11/3
  Gain7/1 -> To Workspace3/1, Mux8/1, dotprod27/2, dotprod6/2, dotprod3/2, Product13/2
  Gain8/1 -> To Workspace2/1, Mux8/2, dotprod2/2, dotprod26/2, dotprod7/2, Product12/2
  Product13/1 -> Mux8/3
  Product12/1 -> Mux8/4
  Product7/1 -> Mux2/4
  Product6/1 -> Mux2/5
  Mux2/1 -> To Workspace5/1, [dW2]
  Mux12/1 -> [dW1], To Workspace7/1
  Mux8/1 -> [dW3], To Workspace12/1
  [dW1] -> Mux11/1
  netsum3/1 -> [wPcmd]
  netsum2/1 -> [vPcmd]
  [B31] -> netsum2/4
  "xref "/1 -> Normalise/1(In1)
  xQ/1 -> Normalise2/1(In1)
  yQ/1 -> Normalise3/1(In1)
  [W222] -> dotprod19/1
  netsum18/1 -> tansig4/1, Mux13/2
  dotprod58/1 -> netsum20/2
  [W212] -> dotprod52/1
  [W242] -> dotprod54/1
  [W122] -> dotprod13/1
  [wref] -> dotprod49/2
  [B22] -> netsum21/5
  [wref] -> dotprod13/2
  [vref] -> dotprod48/2
  dotprod53/1 -> netsum20/1
  [wref] -> dotprod51/2
  dotprod18/1 -> netsum20/3
  [W232] -> dotprod59/1
  [W123] -> dotprod57/1
  dotprod55/1 -> netsum20/4
  [W221] -> dotprod58/1
  netsum23/1 -> tansig2/1, Mux13/4
  netsum22/1 -> tansig6/1, Mux13/1
  [vref] -> dotprod56/2
  [W241] -> dotprod55/1
  [W111] -> dotprod48/1
  [W121] -> dotprod49/1
  dotprod19/1 -> netsum21/2
  [vref] -> dotprod50/2
  [B21] -> netsum20/5
  dotprod54/1 -> netsum21/4
  [W112] -> dotprod12/1
  netsum21/1 -> tansig1/1, Mux9/2
  netsum19/1 -> tansig3/1, Mux13/3
  netsum20/1 -> tansig5/1, Mux9/1
  [W211] -> dotprod53/1
  [W231] -> dotprod18/1
  [B14] -> netsum23/3
  dotprod59/1 -> netsum21/3
  [wref] -> dotprod57/2
  [B13] -> netsum19/3
  [vref] -> dotprod12/2
  [B12] -> netsum18/3
  [W124] -> dotprod51/1
  dotprod52/1 -> netsum21/1
  [W113] -> dotprod56/1
  [W114] -> dotprod50/1
  [B11] -> netsum22/3
  tansig2/1 -> dotprod25/2, dotprod54/2, dotprod55/2, Mux5/4
  tansig3/1 -> Mux5/3, dotprod18/2, dotprod24/2, dotprod59/2
  tansig4/1 -> dotprod23/2, dotprod19/2, dotprod58/2, Mux5/2
  tansig6/1 -> dotprod22/2, dotprod52/2, dotprod53/2, Mux5/1
  dotprod48/1 -> netsum22/1
  dotprod12/1 -> netsum18/1
  dotprod56/1 -> netsum19/1
  dotprod50/1 -> netsum23/1
  dotprod49/1 -> netsum22/2
  dotprod13/1 -> netsum18/2
  dotprod57/1 -> netsum19/2
  dotprod51/1 -> netsum23/2
  dotprod3/1 -> netsum4/1
  dotprod2/1 -> netsum4/2
  Mux13/1 -> dtansig1/1(Z)
  [W221] -> dotprod17/1
  [W212] -> dotprod5/1
  [W241] -> dotprod16/1
  [W242] -> dotprod15/1
  [W232] -> dotprod44/1
  [W222] -> dotprod4/1
  [W231] -> dotprod1/1
  [W211] -> dotprod14/1
  Gain10/1 -> Product15/2
  Gain9/1 -> Product16/2
  netsum6/1 -> Gain9/1
  netsum1/1 -> Gain10/1
  netsum7/1 -> Gain11/1
  Gain11/1 -> Product17/2
  Gain12/1 -> Product18/2
  netsum24/1 -> Gain12/1
  dotprod15/1 -> netsum24/2
  dotprod16/1 -> netsum24/1
  dotprod44/1 -> netsum7/2
  dotprod1/1 -> netsum7/1
  dotprod4/1 -> netsum6/2
  dotprod17/1 -> netsum6/1
  dotprod5/1 -> netsum1/2
  dotprod14/1 -> netsum1/1
  dtansig1/1(Phi) -> Demux4/1
  Demux4/1 -> Product15/1
  Demux4/2 -> Product16/1
  Demux4/3 -> Product17/1
  Demux4/4 -> Product18/1
  From150/1 -> dotprod61/1
  From151/1 -> dotprod62/1
  dotprod64/1 -> netsum26/3
  From148/1 -> dotprod45/1
  dotprod47/1 -> netsum25/1
  dotprod45/1 -> netsum25/2
  From23/1 -> dotprod63/1
  From24/1 -> dotprod64/1
  dotprod63/1 -> netsum25/3
  dotprod60/1 -> netsum26/1
  From112/1 -> dotprod47/1
  netsum25/1 -> Gain14/1
  From22/1 -> dotprod46/1
  dotprod61/1 -> netsum25/4
  From113/1 -> dotprod60/1
  netsum26/1 -> Gain13/1
  dotprod62/1 -> netsum26/4
  dotprod46/1 -> netsum26/2
  Product10/1 -> Mux12/5
  Product1/1 -> Mux12/6
  [W241] -> Mux10/19
  [W212] -> Mux10/20
  [W222] -> Mux10/21
  [W232] -> Mux10/22
  Product15/1 -> Mux3/1
  Product16/1 -> Mux3/2
  Product17/1 -> Mux3/3
  Product18/1 -> Mux3/4
  Mux3/1 -> Product1/2, Product10/2, Demux1/1
  Demux1/1 -> Mux12/1
  Demux1/2 -> Mux12/2
  Demux1/3 -> Mux12/3
  Demux1/4 -> Mux12/4
  [yref] -> Product1/1
  [xref] -> Product10/1
  [W242] -> Mux10/23
  [W213] -> Mux10/24
  [W223] -> Mux10/25
  [W233] -> Mux10/26
  [W243] -> Mux10/27
  [B31] -> Mux10/28
  Mux5/1 -> Product3/1, Product7/1, Product6/1
  Demux3/28 -> [B31]
  Demux3/27 -> [W243]
  Demux3/26 -> [W233]
  Demux3/25 -> [W223]
  Demux3/24 -> [W213]
  Demux3/23 -> [W242]
  Demux3/22 -> [W232]
  Demux3/21 -> [W222]
  Demux3/20 -> [W212]
  Demux3/19 -> [W241]
  yref/1 -> Normalise1/1(In1)
  [W331] -> dotprod20/1
  [W332] -> dotprod21/1
  [B32] -> netsum3/4
  dotprod20/1 -> netsum2/3
  dotprod21/1 -> netsum3/3
  [B23] -> netsum8/5
  [W213] -> dotprod22/1
  dotprod22/1 -> netsum8/1
  [W223] -> dotprod23/1
  dotprod23/1 -> netsum8/2
  [W233] -> dotprod24/1
  dotprod24/1 -> netsum8/3
  [W243] -> dotprod25/1
  dotprod25/1 -> netsum8/4
  Gain1/1 -> Product2/2
  netsum9/1 -> Gain1/1
  [W332] -> dotprod27/1
  [W331] -> dotprod26/1
  dotprod26/1 -> netsum9/1
  dotprod27/1 -> netsum9/2
  Demux/1 -> Product4/1
  Demux/2 -> Product5/1
  netsum8/1 -> Mux9/3, tansig7/1
  Demux/3 -> Product2/1
  [W243] -> dotprod37/1
  Product2/1 -> Mux2/3, Product3/2, dotprod67/2, dotprod66/2, dotprod37/2, dotprod65/2
  dotprod37/1 -> netsum24/3
  [W233] -> dotprod65/1
  dotprod65/1 -> netsum7/3
  [W223] -> dotprod66/1
  dotprod66/1 -> netsum6/3
  [W213] -> dotprod67/1
  dotprod67/1 -> netsum1/3
  Product3/1 -> Mux2/6
  tansig7/1 -> Mux6/3, dotprod20/2, dotprod21/2
  [W332] -> Mux10/35
  [W331] -> Mux10/34
  [W322] -> Mux10/33
  [W321] -> Mux10/32
  [W312] -> Mux10/31
  [B32] -> Mux10/29
  [W311] -> Mux10/30
  Demux3/29 -> [B32]
  Demux3/30 -> [W311]
  Demux3/31 -> [W312]
  Demux3/32 -> [W321]
  Demux3/33 -> [W322]
  Demux3/35 -> [W332]
  Demux3/34 -> [W331]
  Sum17/1 -> Unit Delay1/1, To Workspace1/1
  Mux10/1 -> IC1/1
  Gain2/1 -> Sum17/1
  Unit Delay1/1 -> Demux3/1
  Normalise1/1(Out1) -> [yref], To Workspace6/1
  Normalise/1(Out1) -> To Workspace8/1, [xref]
  Normalise2/1(Out1) -> To Workspace11/1, [xQ]
  Normalise3/1(Out1) -> To Workspace13/1, [yQ]

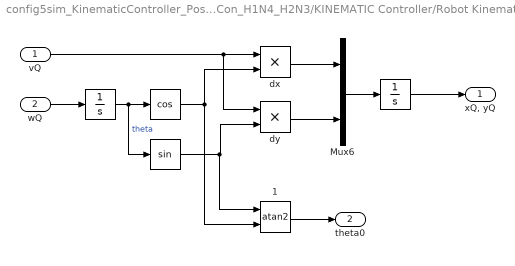
== system config5sim_KinematicController_PosCon_H1N4_H2N3/KINEMATIC Controller/Robot Kinematics ==
  vQ : Inport
  wQ : Inport  Port=2
  " " : Trigonometry  Operator=cos
  "  " : Trigonometry
  "   " : Integrator  InitialCondition=th0
  "    " : Integrator  InitialCondition=[xaxon0 yaxon0]
  "     1" : Trigonometry  Operator=atan2
  Mux6 : Mux  Inputs=2
  dx : Product
  dy : Product
  "xQ, yQ" : Outport  VectorParamsAs1DForOutWhenUnconnected=off
  theta0 : Outport  Port=2  VectorParamsAs1DForOutWhenUnconnected=off
  wires:
  dx/1 -> Mux6/1
  dy/1 -> Mux6/2
  vQ/1 -> dy/1, dx/1
  wQ/1 -> "   "/1
  " "/1 -> "     1"/2, dx/2
  "   "/1 -> "  "/1, " "/1  "theta"
  "  "/1 -> "     1"/1, dy/2
  Mux6/1 -> "    "/1
  "    "/1 -> "xQ, yQ"/1
  "     1"/1 -> theta0/1

== system config5sim_KinematicController_PosCon_H1N4_H2N3/KINEMATIC Controller/Signal Builder ==
  Demux : Demux  Tag=STV Demux  Outputs=3
  FromWs : FromWorkspace  Tag=STV FromWs  VariableName=tuvar  SampleTime=0
      SigBuilderData=|
      | common.afterFinalStr = 'Extrapolate'
      | common.sampleTime = 0
      | dataSet.timeRange = [0 60]
      | dataSet.name = 'Kinematic control parameters'
      | sbobj.Groups.Name = 'Kinematic control parameters'
      | sbobj.Groups.Signals(1).Name = 'k1'
      | sbobj.Groups.Signals(1).XData = [0 6.5 6.5 13.375 13.375 19.875 19.875 26.75 26.75 33.25 33.25 40.125 40.125 46.625 46.625 53.5 53.5 60]
      | sbobj.Groups.Signals(1).YData = [0.8 0.8 0.6 0.6 0.25 0.25 0.3 0.3 0.8 0.8 0.3 0.3 0.25 0.25 0.6 0.6 0.8 0.8]
      | sbobj.Groups.Signals(2).Name = 'k2'
      | sbobj.Groups.Signals(2).XData = [0 6.5 6.5 13.375 13.375 19.875 19.875 26.7379679144 26.75 33.25 33.25 40.125 40.125 46.625 46.625 53.5 53.5 60]
      | sbobj.Groups.Signals(2).YData = [0.1 0.1 2.8 2.8 1.6 1.6 1.8 1.8 0.1 0.1 1.8 1.8 1.6 1.6 2.8 2.8 0.1 0.1]
      | sbobj.Groups.Signals(3).Name = 'k3'
      | sbobj.Groups.Signals(3).XData = [0 6.5 6.5 13.375 13.375 19.875 19.875 26.75 26.75 33.25 33.25 40.125 40.125 46.625 46.625 53.5 53.5 60]
      | sbobj.Groups.Signals(3).YData = [1.5 1.5 2.5 2.5 2 2 5.1 5.1 1.5 1.5 5.1 5.1 2 2 2.5 2.5 1.5 1.5]
      | sbobj.Groups.TimeRange = [0 60]
  k1 : Outport  Tag=STV Outport  VectorParamsAs1DForOutWhenUnconnected=off
  k2 : Outport  Tag=STV Outport  Port=2  VectorParamsAs1DForOutWhenUnconnected=off
  k3 : Outport  Tag=STV Outport  Port=3  VectorParamsAs1DForOutWhenUnconnected=off
  wires:
  Demux/1 -> k1/1
  FromWs/1 -> Demux/1
  Demux/2 -> k2/1
  Demux/3 -> k3/1

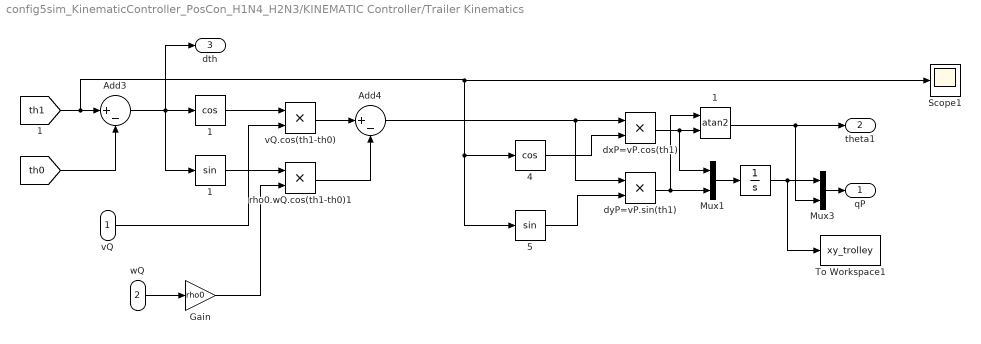
== system config5sim_KinematicController_PosCon_H1N4_H2N3/KINEMATIC Controller/Trailer Kinematics ==
  vQ : Inport
  wQ : Inport  Port=2
  "    " : Integrator  InitialCondition=[xtrolley0 ytrolley0]
  "          1" : Trigonometry
  "         1" : Trigonometry  Operator=cos
  "         4" : Trigonometry  Operator=cos
  "         5" : Trigonometry
  "     1" : Trigonometry  Operator=atan2
  Add3 : Sum  Inputs=|+-
  Add4 : Sum  Inputs=|+-
  Gain : Gain  Gain=rho0
  Mux1 : Mux  Inputs=2
  Mux3 : Mux  Inputs=2
  Scope1 : Scope
  To Workspace1 : ToWorkspace  VariableName=xy_trolley  SaveFormat=Timeseries  SampleTime=-1
  dxP=vP.cos(th1) : Product
  dyP=vP.sin(th1) : Product
  rho0.wQ.cos(th1-th0)1 : Product
  vQ.cos(th1-th0) : Product
  qP : Outport  VectorParamsAs1DForOutWhenUnconnected=off
  theta1 : Outport  Port=2  VectorParamsAs1DForOutWhenUnconnected=off
  dth : Outport  Port=3  VectorParamsAs1DForOutWhenUnconnected=off
  wires:
  "     1"/1 -> theta1/1, Mux3/2
  "    "/1 -> To Workspace1/1, Mux3/1
  vQ.cos(th1-th0)/1 -> Add4/1
  "         1"/1 -> vQ.cos(th1-th0)/1
  Add3/1 -> dth/1, "          1"/1, "         1"/1
  "          1"/1 -> rho0.wQ.cos(th1-th0)1/1
  Gain/1 -> rho0.wQ.cos(th1-th0)1/2
  dyP=vP.sin(th1)/1 -> Mux1/2, "     1"/1
  rho0.wQ.cos(th1-th0)1/1 -> Add4/2
  Mux3/1 -> qP/1
  Mux1/1 -> "    "/1
  vQ/1 -> vQ.cos(th1-th0)/2
  Add4/1 -> dyP=vP.sin(th1)/1, dxP=vP.cos(th1)/1
  dxP=vP.cos(th1)/1 -> "     1"/2, Mux1/1
  wQ/1 -> Gain/1
  [th1] -> Scope1/1, "         5"/1, "         4"/1, Add3/1
  [th0] -> Add3/2
  "         4"/1 -> dxP=vP.cos(th1)/2
  "         5"/1 -> dyP=vP.sin(th1)/2

== system config5sim_KinematicController_PosCon_H1N4_H2N3/KINEMATIC Controller/MLP - NN - WTFITS/Normalise ==
  In1 : Inport
  Constant : Constant  Value=xref_mean
  Constant1 : Constant  Value=xref_std
  Constant2 : Constant  Value=2
  Divide : Product  Inputs=*/
  Sum : Sum  Inputs=|+-
  Out1 : Outport
  wires:
  Constant/1 -> Sum/2
  In1/1 -> Sum/1
  Divide/1 -> Out1/1
  Constant1/1 -> Divide/2
  Sum/1 -> Divide/1

== system config5sim_KinematicController_PosCon_H1N4_H2N3/KINEMATIC Controller/MLP - NN - WTFITS/Normalise1 ==
  In1 : Inport
  Constant : Constant  Value=yref_mean
  Constant1 : Constant  Value=yref_std
  Constant2 : Constant  Value=2
  Divide : Product  Inputs=*/
  Sum : Sum  Inputs=|+-
  Out1 : Outport
  wires:
  Constant/1 -> Sum/2
  In1/1 -> Sum/1
  Divide/1 -> Out1/1
  Constant1/1 -> Divide/2
  Sum/1 -> Divide/1

== system config5sim_KinematicController_PosCon_H1N4_H2N3/KINEMATIC Controller/MLP - NN - WTFITS/Normalise2 ==
  In1 : Inport
  Constant : Constant  Value=2
  Constant1 : Constant  Value=xQ_mean
  Constant2 : Constant  Value=xQ_std
  Divide : Product  Inputs=*/
  Sum : Sum  Inputs=|+-
  Out1 : Outport
  wires:
  Constant1/1 -> Sum/2
  In1/1 -> Sum/1
  Sum/1 -> Divide/1
  Constant2/1 -> Divide/2
  Divide/1 -> Out1/1

== system config5sim_KinematicController_PosCon_H1N4_H2N3/KINEMATIC Controller/MLP - NN - WTFITS/Normalise3 ==
  In1 : Inport
  Constant : Constant  Value=2
  Constant1 : Constant  Value=yQ_std
  Constant2 : Constant  Value=yQ_mean
  Divide : Product  Inputs=*/
  Sum : Sum  Inputs=|+-
  Out1 : Outport
  wires:
  Constant2/1 -> Sum/2
  In1/1 -> Sum/1
  Sum/1 -> Divide/1
  Constant1/1 -> Divide/2
  Divide/1 -> Out1/1

== system config5sim_KinematicController_PosCon_H1N4_H2N3/KINEMATIC Controller/MLP - NN - WTFITS/dtansig ==
  Z : Inport
  Add : Sum  Inputs=+-
  Constant : Constant
  Math Function : Math  Operator=square  SignedPower=off  SaturateOnIntegerOverflow=on
  tansig1 : neural/Transfer Functions/tansig
      settings: SourceProductName=Deep Learning Toolbox
  Phi : Outport
  wires:
  Z/1 -> tansig1/1
  Add/1 -> Phi/1
  Constant/1 -> Add/1
  tansig1/1 -> Math Function/1
  Math Function/1 -> Add/2

== system config5sim_KinematicController_PosCon_H1N4_H2N3/KINEMATIC Controller/MLP - NN - WTFITS/dtansig1 ==
  Z : Inport
  Add : Sum  Inputs=+-
  Constant : Constant
  Math Function : Math  Operator=square  SignedPower=off  SaturateOnIntegerOverflow=on
  tansig1 : neural/Transfer Functions/tansig
      settings: SourceProductName=Deep Learning Toolbox
  Phi : Outport
  wires:
  Z/1 -> tansig1/1
  Add/1 -> Phi/1
  Constant/1 -> Add/1
  tansig1/1 -> Math Function/1
  Math Function/1 -> Add/2
